simulink model "motor"  (R2022b)
settings: Solver=VariableStepAuto  StartTime=0.0  StopTime=3  RelTol=1e-3
values from neighbouring files (symbols this model uses):
  K0 = 1.5    [demo1_tune.m]
  K1 = 1.0    (= 1)    [demo1_tune.m]
  sig0 = 15    [demo1_tune.m]
  sig1 = 10    [demo1_tune.m]
settings Model: Creator=JackPaul  LastModifiedBy=JackPaul

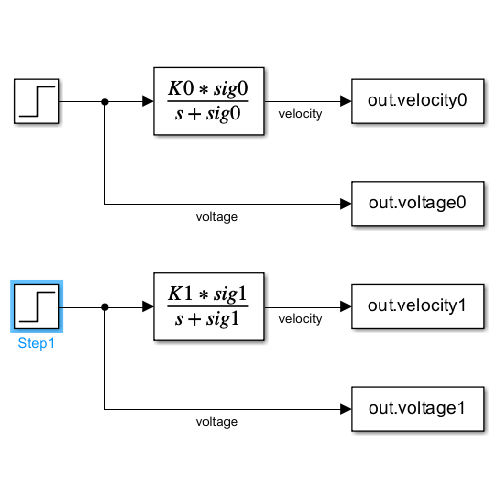
[thumbnail: Simulink's stored preview of the top-level diagram]
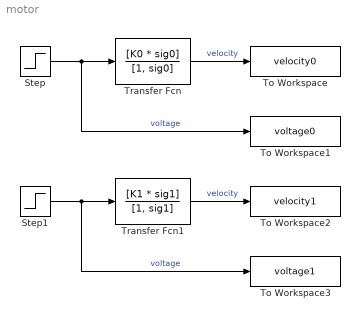
== system motor ==
  Step : Step  After=4  SampleTime=0
  Step1 : Step  After=4  SampleTime=0
  To Workspace : ToWorkspace  VariableName=velocity0  SaveFormat=Timeseries  SampleTime=-1
  To Workspace1 : ToWorkspace  VariableName=voltage0  SaveFormat=Timeseries  SampleTime=-1
  To Workspace2 : ToWorkspace  VariableName=velocity1  SaveFormat=Timeseries  SampleTime=-1
  To Workspace3 : ToWorkspace  VariableName=voltage1  SaveFormat=Timeseries  SampleTime=-1
  Transfer Fcn : TransferFcn  Numerator=[K0 * sig0]  Denominator=[1, sig0]
  Transfer Fcn1 : TransferFcn  Numerator=[K1 * sig1]  Denominator=[1, sig1]
  wires:
  Step/1 -> Transfer Fcn/1, To Workspace1/1  "voltage"
  Transfer Fcn/1 -> To Workspace/1  "velocity"
  Step1/1 -> To Workspace3/1, Transfer Fcn1/1  "voltage"
  Transfer Fcn1/1 -> To Workspace2/1  "velocity"
